simulink model "ClosedLoop_CqCscCi"  (R2023b)
settings: Solver=VariableStepAuto  StartTime=0.0  StopTime=10.0  RelTol=1e-3
libraries: cstblocks x5
settings Model: Creator=Albertlakers  LastModifiedBy=Albertlakers

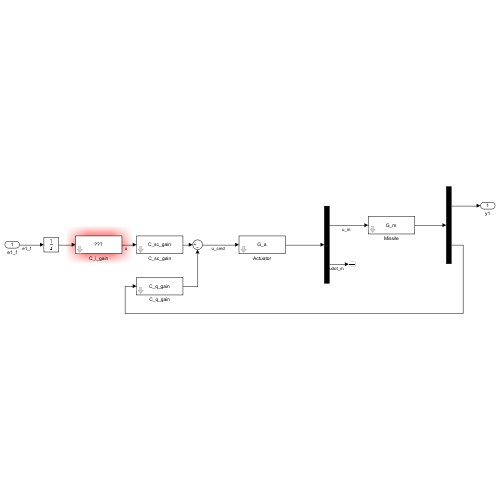
[thumbnail: Simulink's stored preview of the top-level diagram]
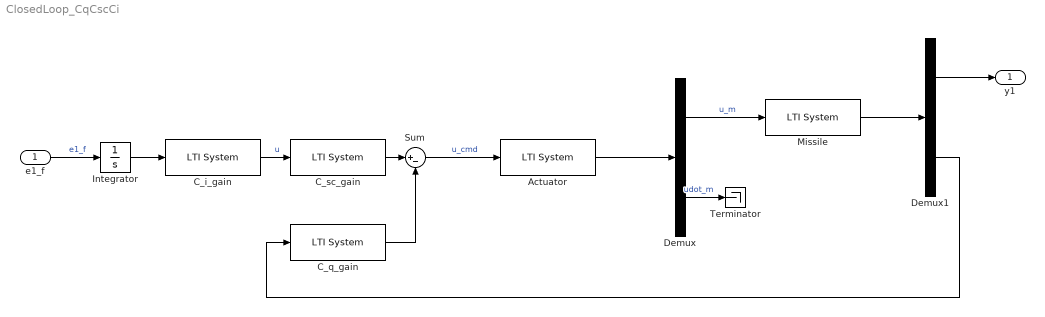
== system ClosedLoop_CqCscCi ==
  e1_f : Inport
  Actuator : cstblocks/LTI System  sys=G_a  IC=[]  PadeOrder=0
  C_i_gain : cstblocks/LTI System  sys=C_i_gain  IC=[]  PadeOrder=0
  C_q_gain : cstblocks/LTI System  sys=C_q_gain  IC=[]  PadeOrder=0
  C_sc_gain : cstblocks/LTI System  sys=C_sc_gain  IC=[]  PadeOrder=0
  Demux : Demux  Outputs=2
  Demux1 : Demux  Outputs=2
  Integrator : Integrator
  Missile : cstblocks/LTI System  sys=G_m  IC=[]  PadeOrder=0
  Sum : Sum  Inputs=|+-
  Terminator : Terminator
  y1 : Outport
  wires:
  Demux/2 -> Terminator/1  "udot_m"
  Demux/1 -> Missile/1  "u_m"
  C_sc_gain/1 -> Sum/1
  Missile/1 -> Demux1/1
  C_q_gain/1 -> Sum/2
  e1_f/1 -> Integrator/1  "e1_f"
  Demux1/2 -> C_q_gain/1
  Sum/1 -> Actuator/1  "u_cmd"
  Demux1/1 -> y1/1
  Actuator/1 -> Demux/1
  Integrator/1 -> C_i_gain/1
  C_i_gain/1 -> C_sc_gain/1  "u"
